simulink model "LCS"  (R2023b)
settings: Solver=VariableStepAuto  StartTime=0.0  StopTime=10.0  RelTol=1e-3
settings Model: Creator=no  LastModifiedBy=no

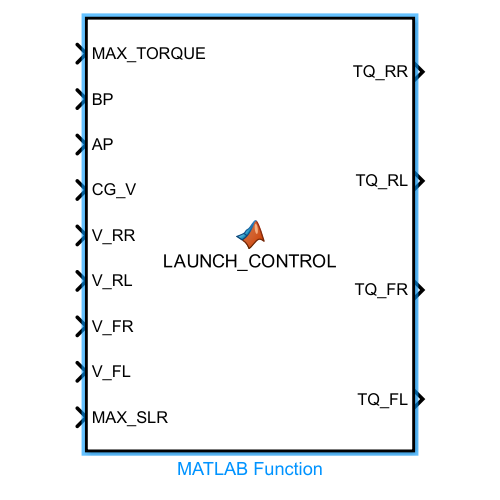
[thumbnail: Simulink's stored preview of the top-level diagram]
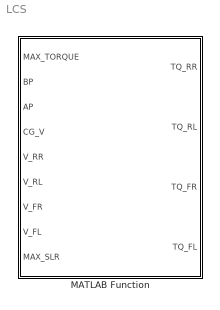
== system LCS ==
  MATLAB Function : MATLAB Function  TreatAsAtomicUnit=on

== matlab function LCS/MATLAB Function ==
  data: MAX_TORQUE input; BP input; AP input; TQ_RR output; CG_V input; V_RR input; V_RL input; V_FR input; V_FL input; TQ_RL output; TQ_FR output; TQ_FL output; MAX_SLR input
function [TQ_RR, TQ_RL, TQ_FR, TQ_FL] = LAUNCH_CONTROL(MAX_TORQUE, BP, AP, CG_V, V_RR, V_RL, V_FR, V_FL, MAX_SLR)
% SLR CALCULATIONS
    % slip ratio rear right wheel
    if(CG_V == 0 || V_RR == 0)
        SLR_RR = 1;
    else
        SLR_RR = (V_RR / CG_V);
    end
    % slip ratio rear left wheel
    if(CG_V == 0 || V_RL == 0)
        SLR_RL = 1;
    else
        SLR_RL = (V_RL / CG_V);
    end
    % slip ratio front right wheel
    if(CG_V == 0 || V_FR == 0)
        SLR_FR = 1;
    else
        SLR_FR = (V_FR / CG_V);
    end
    % slip ratio front left wheel
    if(CG_V == 0 || V_FL == 0)
        SLR_FL = 1;
    else
        SLR_FL = (V_FL / CG_V);
    end

% set up recursive variables for moving torque distribution backwards
    persistent balance % balance = torque% to front axle
    if isempty(balance)
        balance=0.9;
    end
% set up recursive variable for incrementing torque
    persistent torqueR
    if isempty(torqueR)
        torqueR = 0;
    end
    persistent torqueF
    if isempty(torqueF)
        torqueF = 0;
    end
% set up recursive variables for correcting wheelspin
    persistent correctionR % torque correction to the rear axle
    if isempty(correctionR)
        correctionR=0;
    end
    persistent correctionF % torque correction to the front axle
    if isempty(correctionF)
        correctionF=0;
    end
% set LAUNCH bool variable
% end launch if brake is pressed
    persistent launch
    if isempty(launch)
        launch = false;
    end
% define launch start sequence
    if launch == false
        if BP==1 && AP==1
            launch = true; % set launch to true when driver is pressing both pedals fully down
        end
    end
% define sequence stop
if launch==true
    if V_CG > 3 && BP > 0.33 % if driver brakes stop launch sequence
        launch = false;
        torqueR = 0;
        torqueF = torqueR;
        return;
    elseif BP > 0.33
        torqueR = 0;
        torqueF = torqueR;
    end
end
% launch sequence
if launch == true
% look for wheelspin and set corrections
    if max(SLR_FR, SLR_FL) > MAX_SLR
        correctionF = correctionF + 1;
    else
        correctionF = 0;
    end
    if max(SLR_RR, SLR_RL) > MAX_SLR
        correctionR = correctionR + 1;
    else
        correctionF = 0;
    end
% apply torque in the front axle
    if correctionF > 0
        TQ_FR = (torqueF-correctionF);
        TQ_FL = TQ_FR;
    else
        if torqueF < MAX_TORQUE*balance
            torqueF = torqueF + 1;
        end
        TQ_FR = torqueF;
        TQ_FL = TQ_FR;
    end
% apply torque in the rear axle
    if correctionR > 0
        TQ_RR = (torqueR-correctionR);
        TQ_RL = TQ_RR;
    else
        if torqueR < MAX_TORQUE*(1-balance)
            torqueR = torqueR + 1;
        end
        TQ_RR = torqueR;
        TQ_RL = TQ_RR;
    end
% migrate the balance backwards
    if correctionR == 0
        if balance > 0.55
            balance = balance - 0.1;
        end
    end
end
end
